simulink model "Lab2model"  (R2021b)
settings: Solver=VariableStepAuto  StartTime=0.0  StopTime=1  RelTol=1e-3
values from neighbouring files (symbols this model uses):
  J = moment_of_inertia_after_gear_box    (= 0.002369664)    [Lab_2.m]
  Ke = (KeN+KeP) / 2    [Lab_2.m]
  Km = Ke    [Lab_2.m]
  L = 0.0047    [Lab_2.m]
  R = resistance    [Lab_2.m]
  U = voltages(i)    [Lab_2.m]
settings Model: Creator=romas  LastModifiedBy=huynh

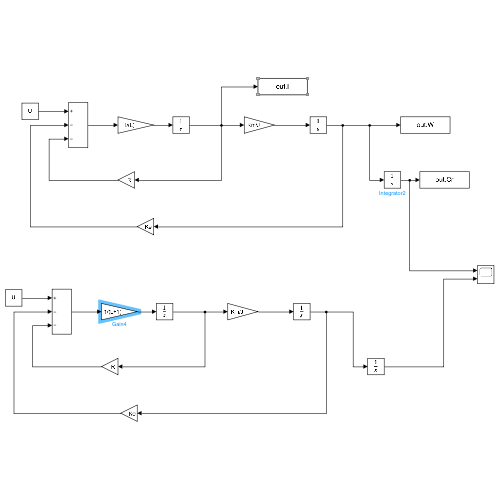
[thumbnail: Simulink's stored preview of the top-level diagram]
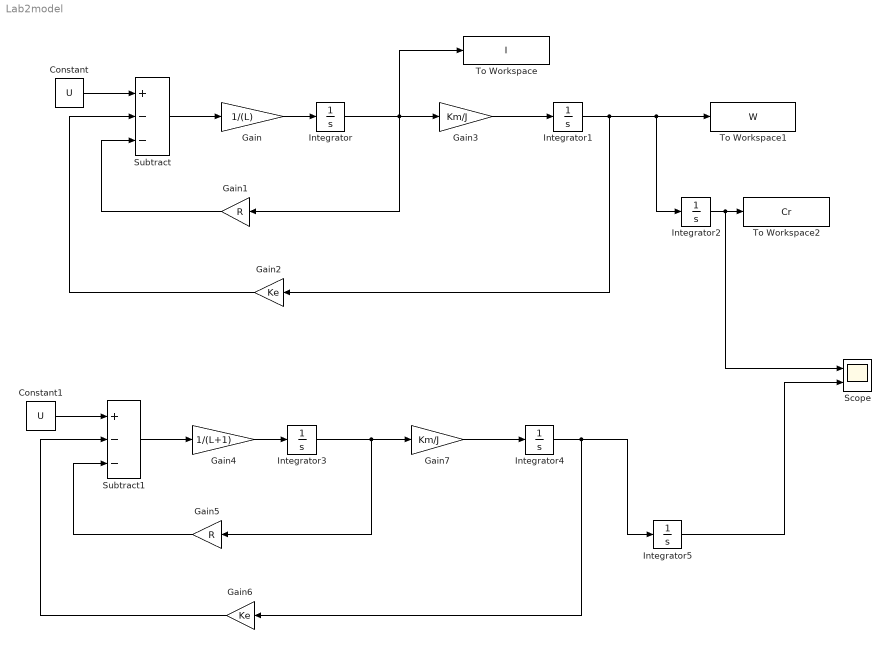
== system Lab2model ==
  Constant : Constant  Value=U
  Constant1 : Constant  Value=U
  Gain : Gain  Gain=1/(L)
  Gain1 : Gain  Gain=R
  Gain2 : Gain  Gain=Ke
  Gain3 : Gain  Gain=Km/J
  Gain4 : Gain  Gain=1/(L+1)
  Gain5 : Gain  Gain=R
  Gain6 : Gain  Gain=Ke
  Gain7 : Gain  Gain=Km/J
  Integrator{,1..5} (6 alike) : Integrator
  Scope : Scope  NumInputPorts=2
  Subtract : Sum  Inputs=+--
  Subtract1 : Sum  Inputs=+--
  To Workspace : ToWorkspace  VariableName=I  SaveFormat=Timeseries  SampleTime=-1
  To Workspace1 : ToWorkspace  VariableName=W  SaveFormat=Timeseries  SampleTime=-1
  To Workspace2 : ToWorkspace  VariableName=Cr  SaveFormat=Timeseries  SampleTime=-1
  wires:
  Constant/1 -> Subtract/1
  Subtract/1 -> Gain/1
  Gain/1 -> Integrator/1
  Gain2/1 -> Subtract/2
  Gain1/1 -> Subtract/3
  Integrator/1 -> Gain3/1, Gain1/1, To Workspace/1
  Gain3/1 -> Integrator1/1
  Integrator1/1 -> Gain2/1, Integrator2/1, To Workspace1/1
  Integrator2/1 -> Scope/1, To Workspace2/1
  Constant1/1 -> Subtract1/1
  Integrator4/1 -> Gain6/1, Integrator5/1
  Gain7/1 -> Integrator4/1
  Integrator3/1 -> Gain7/1, Gain5/1
  Gain6/1 -> Subtract1/2
  Gain4/1 -> Integrator3/1
  Subtract1/1 -> Gain4/1
  Gain5/1 -> Subtract1/3
  Integrator5/1 -> Scope/2
